simulink model "RobotArm"  (R2020a)
settings: Solver=FixedStepAuto  StartTime=0.0  StopTime=2  FixedStep=0.0000001  RelTol=1e-1
libraries: simulink x2
settings Model: SimulationMode=accelerator  Creator=nikhil  LastModifiedBy=nikhil

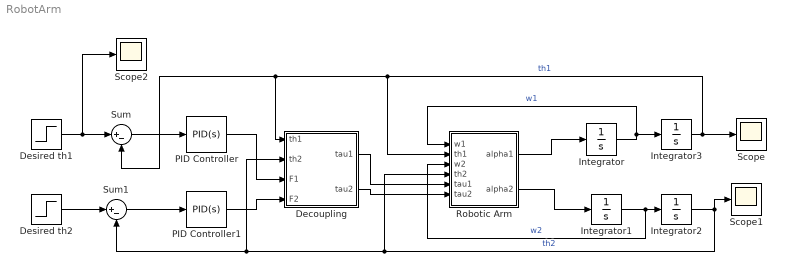
== system RobotArm ==
  Decoupling : Subsystem
  Desired th1 : Step  Time=0  After=0.25*pi  SampleTime=0
  Desired th2 : Step  Time=0  After=1.75*pi  SampleTime=0
  Integrator : Integrator  InitialCondition=0.1  UpperSaturationLimit=10000  LowerSaturationLimit=-10000
  Integrator1 : Integrator  InitialCondition=0.1  UpperSaturationLimit=10000  LowerSaturationLimit=-10000
  Integrator2 : Integrator  InitialCondition=0.001  UpperSaturationLimit=10000  LowerSaturationLimit=-10000
  Integrator3 : Integrator  InitialCondition=0.001  UpperSaturationLimit=10000  LowerSaturationLimit=-10000
  PID Controller : simulink/Continuous/PID Controller  Controller=PID  Form=Parallel  TimeDomain=Continuous-time  UseExternalTs=off  SampleTime=-1  IntegratorMethod=Forward Euler  FilterMethod=Forward Euler  ControllerParametersSource=internal  P=293858.205880481  I=61.6368609867997  D=0.00360479405577455  UseFilter=on  N=1207425.22561184  TunerSelectOption=Transfer Function Based (PID Tuner App)  InitialConditionSource=internal  InitialConditionForIntegrator=0.001  InitialConditionForFilter=0  DifferentiatorICPrevScaledInput=0.001  ExternalReset=none  TrackingMode=off  Kt=1  LimitOutput=off  UpperSaturationLimit=100  LowerSaturationLimit=-100  LinearizeAsGain=on  AntiWindupMode=none  Kb=1  POutMin=[]  POutMax=[]  IOutMin=[]  IOutMax=[]  DOutMin=[]  DOutMax=[]  NOutMin=[]  NOutMax=[]  SumOutMin=[]  SumOutMax=[]  SaturationOutMin=[]  SaturationOutMax=[]  PParamMin=[]  PParamMax=[]  IParamMin=[]  IParamMax=[]  DParamMin=[]  DParamMax=[]  NParamMin=[]  NParamMax=[]  KbParamMin=[]  KbParamMax=[]  KtParamMin=[]  KtParamMax=[]  KbOutMin=[]  KbOutMax=[]  KtOutMin=[]  KtOutMax=[]  IntegratorOutMin=[]  IntegratorOutMax=[]  FilterOutMin=[]  FilterOutMax=[]  SumI1OutMin=[]  SumI1OutMax=[]  SumI2OutMin=[]  SumI2OutMax=[]  SumI3OutMin=[]  SumI3OutMax=[]  SumI4OutMin=[]  SumI4OutMax=[]  SumDOutMin=[]  SumDOutMax=[]  DifferentiatorOutMin=[]  DifferentiatorOutMax=[]  FilterDiffOutCoefMin=[]  FilterDiffOutCoefMax=[]  ReciprocalOutMin=[]  ReciprocalOutMax=[]  SumDenOutMin=[]  SumDenOutMax=[]  SumNumOutMin=[]  SumNumOutMax=[]  DivideOutMin=[]  DivideOutMax=[]  UdiffTsProdOutMin=[]  UdiffTsProdOutMax=[]  NTsProdOutMin=[]  NTsProdOutMax=[]  UintegralTsProdOutMin=[]  UintegralTsProdOutMax=[]  UngainTsProdOutMin=[]  UngainTsProdOutMax=[]  IntegratorContinuousStateAttributes=''  IntegratorStateMustResolveToSignalObject=off  IntegratorRTWStateStorageClass=Auto  FilterContinuousStateAttributes=''  FilterStateMustResolveToSignalObject=off  FilterRTWStateStorageClass=Auto  ParallelPVariant=InternalParameters  IdealPVariant=Disabled  IVariant=InternalParameters  DVariant=InternalParameters  IntegratorVariant=Continuous  SatVariant=Disabled  AWVariant=Passthrough  PCopyVariant=Disabled  TRVariant=Disabled  FdbkBlocksVariant=Forward  IdealPFdbkVariant=Disabled  SatFdbkVariant=Disabled  DerivativeFilterVariant=ContFilter  NVariant=InternalParameters  NCopyVariant=Disabled  FilterICVariant=InternalICsFilter  IntegratorICVariant=InternalICs  ExternalResetVariant=Disabled  TRSumVariant=Passthrough  SumFdbkVariant=Disabled  SumVariant=Sum_PID  TsampFilterVariant=InternalTs  TsampNgainVariant=Passthrough  TsampIntegralVariant=Passthrough
  PID Controller1 : simulink/Continuous/PID Controller  Controller=PID  Form=Parallel  TimeDomain=Continuous-time  UseExternalTs=off  SampleTime=-1  IntegratorMethod=Forward Euler  FilterMethod=Forward Euler  ControllerParametersSource=internal  P=-914264.309564234  I=544.811597799765  D=0.000430068924460639  UseFilter=on  N=100956.534986007  TunerSelectOption=Transfer Function Based (PID Tuner App)  InitialConditionSource=internal  InitialConditionForIntegrator=0.001  InitialConditionForFilter=0  DifferentiatorICPrevScaledInput=0.1  ExternalReset=none  TrackingMode=off  Kt=1  LimitOutput=off  UpperSaturationLimit=100  LowerSaturationLimit=-100  LinearizeAsGain=on  AntiWindupMode=none  Kb=1  SaturateOnIntegerOverflow=on  POutMin=[]  POutMax=[]  IOutMin=[]  IOutMax=[]  DOutMin=[]  DOutMax=[]  NOutMin=[]  NOutMax=[]  SumOutMin=[]  SumOutMax=[]  SaturationOutMin=[]  SaturationOutMax=[]  PParamMin=[]  PParamMax=[]  IParamMin=[]  IParamMax=[]  DParamMin=[]  DParamMax=[]  NParamMin=[]  NParamMax=[]  KbParamMin=[]  KbParamMax=[]  KtParamMin=[]  KtParamMax=[]  KbOutMin=[]  KbOutMax=[]  KtOutMin=[]  KtOutMax=[]  IntegratorOutMin=[]  IntegratorOutMax=[]  FilterOutMin=[]  FilterOutMax=[]  SumI1OutMin=[]  SumI1OutMax=[]  SumI2OutMin=[]  SumI2OutMax=[]  SumI3OutMin=[]  SumI3OutMax=[]  SumI4OutMin=[]  SumI4OutMax=[]  SumDOutMin=[]  SumDOutMax=[]  DifferentiatorOutMin=[]  DifferentiatorOutMax=[]  FilterDiffOutCoefMin=[]  FilterDiffOutCoefMax=[]  ReciprocalOutMin=[]  ReciprocalOutMax=[]  SumDenOutMin=[]  SumDenOutMax=[]  SumNumOutMin=[]  SumNumOutMax=[]  DivideOutMin=[]  DivideOutMax=[]  UdiffTsProdOutMin=[]  UdiffTsProdOutMax=[]  NTsProdOutMin=[]  NTsProdOutMax=[]  UintegralTsProdOutMin=[]  UintegralTsProdOutMax=[]  UngainTsProdOutMin=[]  UngainTsProdOutMax=[]  IntegratorContinuousStateAttributes=''  IntegratorStateMustResolveToSignalObject=off  IntegratorRTWStateStorageClass=Auto  FilterContinuousStateAttributes=''  FilterStateMustResolveToSignalObject=off  FilterRTWStateStorageClass=Auto  ParallelPVariant=InternalParameters  IdealPVariant=Disabled  IVariant=InternalParameters  DVariant=InternalParameters  IntegratorVariant=Continuous  SatVariant=Disabled  AWVariant=Passthrough  PCopyVariant=Disabled  TRVariant=Disabled  FdbkBlocksVariant=Forward  IdealPFdbkVariant=Disabled  SatFdbkVariant=Disabled  DerivativeFilterVariant=ContFilter  NVariant=InternalParameters  NCopyVariant=Disabled  FilterICVariant=InternalICsFilter  IntegratorICVariant=InternalICs  ExternalResetVariant=Disabled  TRSumVariant=Passthrough  SumFdbkVariant=Disabled  SumVariant=Sum_PID  TsampFilterVariant=InternalTs  TsampNgainVariant=Passthrough  TsampIntegralVariant=Passthrough
  Robotic Arm : Subsystem
  Scope : Scope
  Scope1 : Scope
  Scope2 : Scope
  Sum : Sum  Inputs=|+-
  Sum1 : Sum  Inputs=|+-
  wires:
  Integrator1/1 -> Robotic Arm/3(w2), Integrator2/1  "w2"
  Desired th1/1 -> Scope2/1, Sum/1
  Desired th2/1 -> Sum1/1
  Robotic Arm/1(alpha1) -> Integrator/1
  Integrator/1 -> Robotic Arm/1(w1), Integrator3/1  "w1"
  Robotic Arm/2(alpha2) -> Integrator1/1
  Integrator2/1 -> Robotic Arm/4(th2), Decoupling/2(th2), Sum1/2, Scope1/1  "th2"
  Integrator3/1 -> Robotic Arm/2(th1), Decoupling/1(th1), Sum/2, Scope/1  "th1"
  Decoupling/1(tau1) -> Robotic Arm/5(tau1)
  Decoupling/2(tau2) -> Robotic Arm/6(tau2)
  PID Controller/1 -> Decoupling/3(F1)
  PID Controller1/1 -> Decoupling/4(F2)
  Sum/1 -> PID Controller/1
  Sum1/1 -> PID Controller1/1

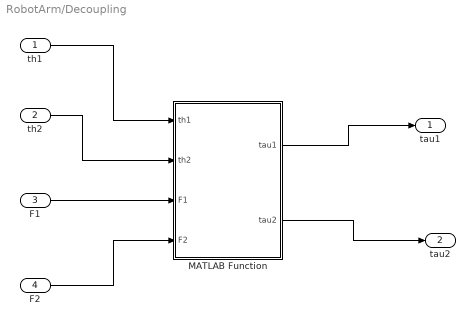
== system RobotArm/Decoupling ==
  th1 : Inport
  th2 : Inport  Port=2
  F1 : Inport  Port=3
  F2 : Inport  Port=4
  MATLAB Function : MATLAB Function  TreatAsAtomicUnit=on
  tau1 : Outport
  tau2 : Outport  Port=2
  wires:
  th1/1 -> MATLAB Function/1(th1)
  th2/1 -> MATLAB Function/2(th2)
  F1/1 -> MATLAB Function/3(F1)
  F2/1 -> MATLAB Function/4(F2)
  MATLAB Function/1(tau1) -> tau1/1
  MATLAB Function/2(tau2) -> tau2/1

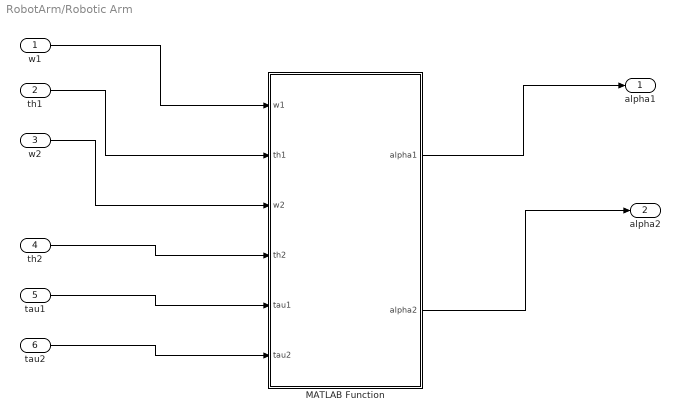
== system RobotArm/Robotic Arm ==
  w1 : Inport
  th1 : Inport  Port=2
  w2 : Inport  Port=3
  th2 : Inport  Port=4
  tau1 : Inport  Port=5
  tau2 : Inport  Port=6
  MATLAB Function : MATLAB Function  TreatAsAtomicUnit=on
  alpha1 : Outport
  alpha2 : Outport  Port=2
  wires:
  w1/1 -> MATLAB Function/1(w1)
  th1/1 -> MATLAB Function/2(th1)
  w2/1 -> MATLAB Function/3(w2)
  th2/1 -> MATLAB Function/4(th2)
  tau1/1 -> MATLAB Function/5(tau1)
  tau2/1 -> MATLAB Function/6(tau2)
  MATLAB Function/1(alpha1) -> alpha1/1
  MATLAB Function/2(alpha2) -> alpha2/1

== matlab function RobotArm/Robotic Arm/MATLAB Function ==
  data: w1 input; alpha1 output; th1 input; w2 input; th2 input; tau1 input; tau2 input; alpha2 output
function [alpha1,alpha2] = fcn(w1,th1,w2,th2,tau1,tau2)
    m1=1;
    m2=1;
    l1=0.2;
    l2=0.2;
    g=9.81;
    
    alpha2 = (tau2*((m1+m2)*l1^2 + m2*l2^2 + 2*m2*l1*l2*cos(th2))+(-m2*l1*l2*sin(th2)*(w1^2)-m2*g*l2*sin(th1+th2))*((m1+m2)*(l1^2) +m2*(l2^2) + 2*m2*l1*l2*cos(th2))-tau1*(m2*(l2^2)+ m2*l1*l2*cos(th2))-(2*m2*l1*l2*sin(th2)*w1*w2 + m2*l1*l2*sin(th2)*(w2^2)-(m1+m2)*g*l1*sin(th1)-m2*g*l2*sin(th1+th2))*(m2*(l2^2)+m2*l1*l2*cos(th2)))/((m2*(l2^2))*((m1+m2)*(l1^2)+m2*(l2^2)+2*m1*l1*l2*cos(th2))-(m2*(l2^2)+m2*l1*l2*cos(th2))^2);
    
    alpha1 = (tau1 - ((m2*l2^2 + m2*l1*l2*cos(th2))*alpha2+2*m2*l1*l2*sin(th2)*w1*w2 + m2*l1*l2*sin(th2)*w2^2-(m1+m2)*g*l1*sin(th1)-m2*g*l2*sin(th1+th2)))/((m1+m2)*(l1^2)+m2*(l2^2)+2*m2*l1*l2*cos(th2));

== matlab function RobotArm/Decoupling/MATLAB Function ==
  data: th1 input; tau1 output; th2 input; F1 input; F2 input; tau2 output
function [tau1,tau2] = fcn(th1, th2, F1, F2)
   l1 = 0.2;
   l2 = 0.2;
   J = [l2*cos(th1+th2)+l1*cos(th1), l2*cos(th1+th2);
         l2*sin(th1+th2)+l1*sin(th1), l2*sin(th1+th2)];
   tau1 = J(1,1)*F1 + J(1,2)*F2;
   tau2 = J(2,1)*F1 + J(2,2)*F2;
